simulink model "SlideMode_Control"  (R2021b)
settings: Solver=ode1  StartTime=0.0  StopTime=220  FixedStep=0.01  RelTol=1e-3
values from neighbouring files (symbols this model uses):
  AirDensity_kgpm3 = 1.225    [vehicle_controller.mat]
  BatteryCapacity_Wh = 83    [vehicle_controller.mat]
  BatteryInitialEnergy = 58.1    [vehicle_controller.mat]
  BatteryMaxVoltage_V = 96    [vehicle_controller.mat]
  BatteryVoltageCoefficient_x = [0 0.1 0.2 0.3 0.4 0.5 0.6 0.7 0.8 0.9 1]    [vehicle_controller.mat]
  BatteryVoltageCoefficient_y = [0.833333333333 0.85 0.866666666667 0.883333333333 0.9 0.916666666667 0.933333333333 0.95 0.966666666667 0.983333333333 1]    [vehicle_controller.mat]
  BodyInitialSpeed_mps = 0    [vehicle_controller.mat]
  BodyMass_kg = 900    [vehicle_controller.mat]
  CombustionEngineMaxTorque_Nm = 100    [vehicle_controller.mat]
  DragArea_m2 = 4.5    [vehicle_controller.mat]
  DragCoeficient_1 = 0.4    [vehicle_controller.mat]
  FrictionCoefficient_Nsprad = 0.01    [vehicle_controller.mat]
  GearboxRatio_0_1 = 3    [vehicle_controller.mat]
  Ke = 0.1178    [vehicle_controller.mat]
  Kt = 0.668    [vehicle_controller.mat]
  L = looptransfer.Lo    [H_infinity_control_design.m]    (also in LoopShaping.m = G*K; Vehicle_Car_Controller.m = P * C)
  R = 0.141176    [vehicle_controller.mat]
  WheelDiameter_m = 0.5    [vehicle_controller.mat]
libraries: simulink x11, simulink_extras x1, cstblocks x1
settings Model: Creator=beni  LastModifiedBy=beni
settings SolverCC: ZeroCrossAlgorithm=Adaptive
settings DataIOCC: ReturnWorkspaceOutputs=off
settings DebuggingCC: IgnoredZcDiagnostic=none

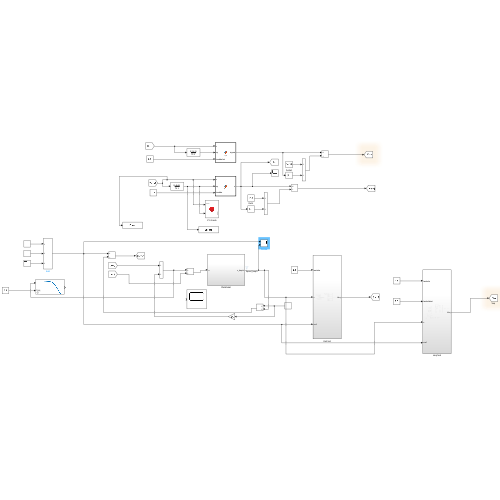
[thumbnail: Simulink's stored preview of the top-level diagram]
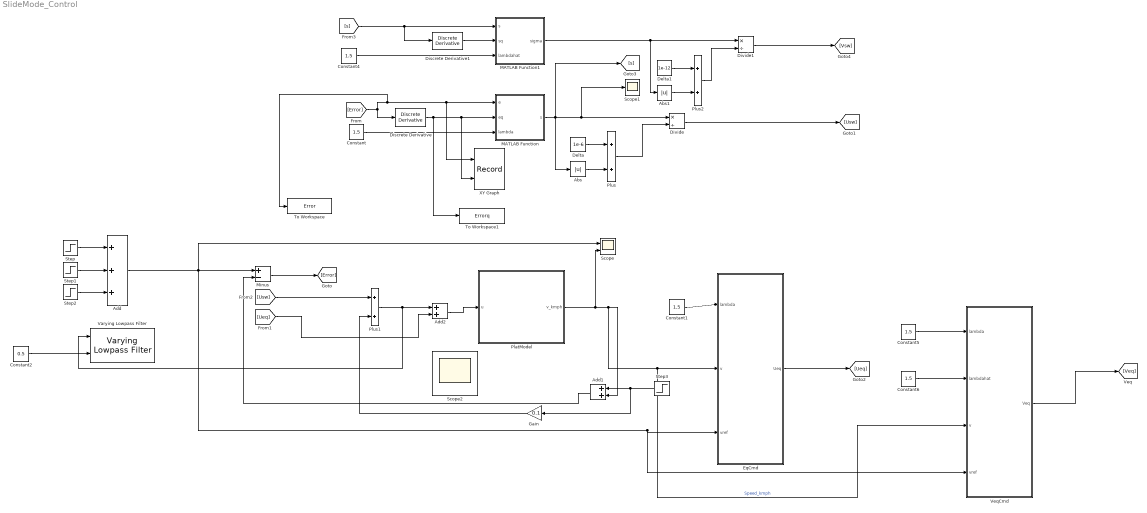
== system SlideMode_Control ==
  Abs : Abs
  Abs1 : Abs
  Add : Sum  Inputs=+++
  Add1 : Sum
  Add2 : Sum
  Constant{,1,4..6} (5 alike) : Constant  Value=1.5
  Constant2 : Constant  Value=0.5
  Delta : Constant  Value=1e-6
  Delta1 : Constant  Value=1e-12
  Discrete Derivative : simulink/Discrete/Discrete Derivative  gainval=1.0  ICPrevScaledInput=0.0  OutMin=[]  OutMax=[]  OutDataType=fixdt(1, 16)  OutScaling=2^-10  DoSatur=off
  Discrete Derivative1 : simulink/Discrete/Discrete Derivative  gainval=1.0  ICPrevScaledInput=0.0  OutMin=[]  OutMax=[]  OutDataType=fixdt(1, 16)  OutScaling=2^-10  DoSatur=off
  Divide : Product  Inputs=*/
  Divide1 : Product  Inputs=*/
  EqCmd : Subsystem
  Gain : Gain  Gain=0.1
  MATLAB Function : MATLAB Function  TreatAsAtomicUnit=on
  MATLAB Function1 : MATLAB Function  TreatAsAtomicUnit=on
  Minus : Sum  Inputs=+-
  PlatModel : Subsystem
  Plus : Sum
  Plus1 : Sum
  Plus2 : Sum
  Scope : Scope  NumInputPorts=2
  Scope1 : Scope
  Scope2 : Scope
  Step : Step  After=63  SampleTime=0
  Step1 : Step  Time=100  After=75  SampleTime=0
  Step2 : Step  Time=150  After=-20  SampleTime=0
  Step3 : Step  Time=40  After=5  SampleTime=0
  To Workspace : ToWorkspace  VariableName=Error  SampleTime=-1
  To Workspace1 : ToWorkspace  VariableName=Errorq  SampleTime=-1
  Varying Lowpass Filter : cstblocks/Linear Parameter Varying/Varying Lowpass Filter  N=1
  VeqCmd : Subsystem
  XY Graph : Record  FileSettingsInternal="{\"entries\":[{\"content\":{\"excelSettings\":{\"content\":{},\"type\":\"Streamout.ExcelSettings\"}},\"type\":\"Streamout.FileSettingStorage\",\"uuid\":\"e4c54855-29c5-47fe-8363-1f54683a9ba0\"}],\"packageUris\":[\"http://schema.mathworks.com/mf0/streamout_blocks/R2020a\"],\"version\":\"1.0\"}"  Layout=[1 1]  SignalsInternal="{\"entries\":[{\"content\":{\"signals\":[{\"content\":{\"blockPath\":[\"SlideMode_Control/XY Graph\"],\"channel\":[],\"dimensions\":[1],\"domain\":\"SlideMode_Control/XY Graph\",\"lineColor\":\"#a2142f\",\"plots\":[],\"port\":1,\"sid\":[\"\"],\"signalID\":7298,\"signalName\":\"From\"},\"type\":\"RecordBlkView.Signal\",\"uuid\":\"8499915c-e861-4faa-950b-0bc3fc22a372\"},{\"content\":{\"blockPath\":[\"SlideMode_Control/XY Graph\"],\"channel\":[],\"dimensions\":[1],\"domain\":\"SlideMode_Control/XY Graph\",\"lineColor\":\"#139fff\",\"plots\":[1],\"port\":2,\"sid\":[\"\"],\"signalID\":7302,\"signalName\":\"Discrete Derivative\"},\"type\":\"RecordBlkView.Signal\",\"uuid\":\"a22b5c38-c1a7-44f1-81eb-330b2b590f18\"}]},\"type\":\"RecordBlkView.InputSignals\",\"uuid\":\"09383715-5c63-4da3-889c-474507ecce84\"}],\"packageUris\":[\"http://schema.mathworks.com/mf0/streamout_blocks/R2020a\"],\"version\":\"1.0\"}"  VisualizationBindings="{\"xyplotplugin\":{\"info\":[{\"series\":[{\"bindingParametersList\":[{\"parameter\":\"Y-Axis\",\"signalID\":7302,\"signalName\":\"Discrete Derivative\"}],\"seriesID\":63923}],\"subplotID\":1}]}}"  CompatibilityTag=XY
  wires:
  PlatModel/1(v_kmph) -> Scope/2, Add1/2, VeqCmd/3(v), EqCmd/2(v)  "Speed_kmph"
  Minus/1 -> [Error]
  [Error] -> Discrete Derivative/1, To Workspace/1, XY Graph/1, MATLAB Function/1(e)
  Discrete Derivative/1 -> To Workspace1/1, XY Graph/2, MATLAB Function/2(eq)
  Constant/1 -> MATLAB Function/3(lambda)
  Abs/1 -> Plus/2
  MATLAB Function/1(s) -> [s], Scope1/1, Divide/1, Abs/1
  Delta/1 -> Plus/1
  Plus/1 -> Divide/2
  Constant1/1 -> EqCmd/1(lambda)
  EqCmd/1(Ueq) -> [Ueq]
  [Usw] -> Plus1/1
  Divide/1 -> [Usw]
  Constant2/1 -> Varying Lowpass Filter/2
  VeqCmd/1(Veq) -> [Veq]
  Discrete Derivative1/1 -> MATLAB Function1/2(sq)
  [s] -> Discrete Derivative1/1, MATLAB Function1/1(s)
  Constant4/1 -> MATLAB Function1/3(lambdahat)
  Delta1/1 -> Plus2/1
  Plus2/1 -> Divide1/2
  MATLAB Function1/1(sigma) -> Abs1/1, Divide1/1
  Divide1/1 -> [Vsw]
  Abs1/1 -> Plus2/2
  Constant5/1 -> VeqCmd/1(lambda)
  Constant6/1 -> VeqCmd/2(lambdahat)
  Plus1/1 -> Add2/1, Varying Lowpass Filter/1
  Add/1 -> Scope/1, VeqCmd/4(vref), EqCmd/3(vref), Minus/1
  Add1/1 -> Minus/2
  Step/1 -> Add/1
  Step1/1 -> Add/2
  Step2/1 -> Add/3
  Step3/1 -> Gain/1, Add1/1
  Add2/1 -> PlatModel/1(u)
  Gain/1 -> Plus1/2
  [Ueq] -> Add2/2

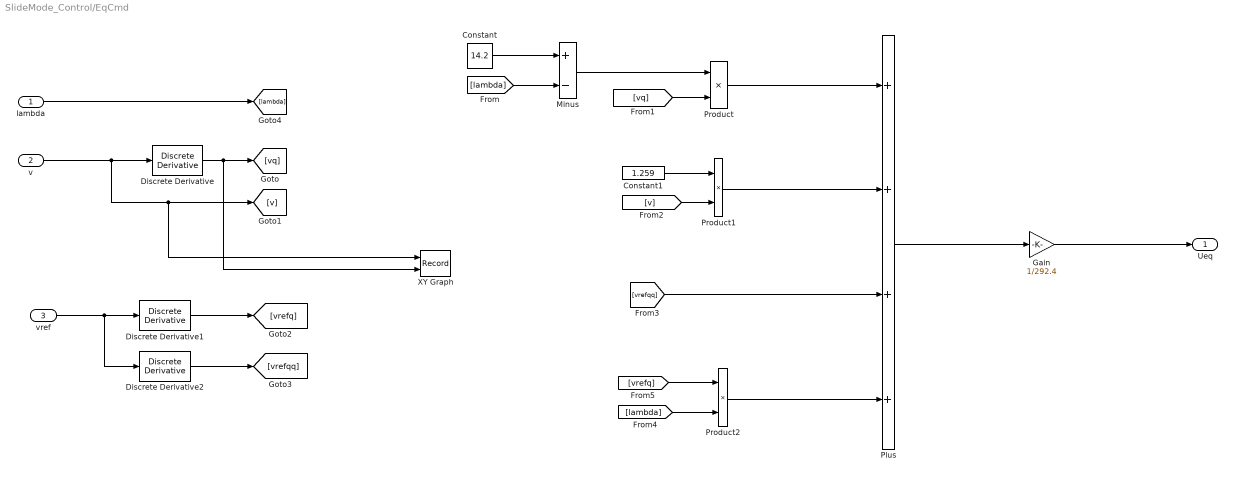
== system SlideMode_Control/EqCmd ==
  lambda : Inport
  v : Inport  Port=2
  vref : Inport  Port=3
  Constant : Constant  Value=14.2
  Constant1 : Constant  Value=1.259
  Discrete Derivative : simulink/Discrete/Discrete Derivative  gainval=1.0  ICPrevScaledInput=0.0  OutMin=[]  OutMax=[]  OutDataType=fixdt(1, 16)  OutScaling=2^-10  DoSatur=off
  Discrete Derivative1 : simulink/Discrete/Discrete Derivative  gainval=1.0  ICPrevScaledInput=0.0  OutMin=[]  OutMax=[]  OutDataType=fixdt(1, 16)  OutScaling=2^-10  DoSatur=off
  Discrete Derivative2 : simulink/Discrete/Discrete Derivative  gainval=1.0  ICPrevScaledInput=0.0  OutMin=[]  OutMax=[]  OutDataType=fixdt(1, 16)  OutScaling=2^-10  DoSatur=off
  Gain : Gain  Gain=1/292.4
  Minus : Sum  Inputs=+-
  Plus : Sum  Inputs=++++
  Product : Product
  Product1 : Product
  Product2 : Product
  XY Graph : Record  FileSettingsInternal="{\"entries\":[{\"content\":{\"excelSettings\":{\"content\":{},\"type\":\"Streamout.ExcelSettings\"}},\"type\":\"Streamout.FileSettingStorage\",\"uuid\":\"b16a5f91-d4a1-49a2-a27a-15ddc10f0a7e\"}],\"packageUris\":[\"http://schema.mathworks.com/mf0/streamout_blocks/R2020a\"],\"version\":\"1.0\"}"  Layout=[1 1]  SignalsInternal="{\"entries\":[{\"content\":{\"signals\":[{\"content\":{\"blockPath\":[\"SlideMode_Control/EqCmd/XY Graph\"],\"channel\":[],\"dimensions\":[1],\"domain\":\"SlideMode_Control/EqCmd/XY Graph\",\"lineColor\":\"#a2142f\",\"plots\":[1],\"port\":1,\"sid\":[\"\"],\"signalID\":7314,\"signalName\":\"v\"},\"type\":\"RecordBlkView.Signal\",\"uuid\":\"f1ec4534-eb6a-4768-bd96-3897fc4c94d6\"},{\"content\":{\"blockPath\":[\"SlideMode_Control/EqCmd/XY Graph\"],\"channel\":[],\"dimensions\":[1],\"domain\":\"SlideMode_Control/EqCmd/XY Graph\",\"lineColor\":\"#139fff\",\"plots\":[1],\"port\":2,\"sid\":[\"\"],\"signalID\":7318,\"signalName\":\"Discrete Derivative\"},\"type\":\"RecordBlkView.Signal\",\"uuid\":\"f4cb1554-1745-48c5-b1b8-53c7b26e64ab\"}]},\"type\":\"RecordBlkView.InputSignals\",\"uuid\":\"a4abee9c-6360-49de-9ab9-487291d355fa\"}],\"packageUris\":[\"http://schema.mathworks.com/mf0/streamout_blocks/R2020a\"],\"version\":\"1.0\"}"  VisualizationBindings="{\"xyplotplugin\":{\"info\":[{\"series\":[{\"bindingParametersList\":[{\"parameter\":\"X-Axis\",\"signalID\":7314,\"signalName\":\"v\"},{\"parameter\":\"Y-Axis\",\"signalID\":7318,\"signalName\":\"Discrete Derivative\"}],\"seriesID\":11742}],\"subplotID\":1}]}}"  CompatibilityTag=XY
  Ueq : Outport
  wires:
  v/1 -> Discrete Derivative/1, XY Graph/1, [v]
  Discrete Derivative/1 -> XY Graph/2, [vq]
  vref/1 -> Discrete Derivative2/1, Discrete Derivative1/1
  Discrete Derivative1/1 -> [vrefq]
  Discrete Derivative2/1 -> [vrefqq]
  lambda/1 -> [lambda]
  Constant/1 -> Minus/1
  [lambda] -> Minus/2
  Minus/1 -> Product/1
  [vq] -> Product/2
  Product/1 -> Plus/1
  Constant1/1 -> Product1/1
  [v] -> Product1/2
  Product1/1 -> Plus/2
  [vrefqq] -> Plus/3
  Product2/1 -> Plus/4
  [lambda] -> Product2/2
  [vrefq] -> Product2/1
  Plus/1 -> Gain/1
  Gain/1 -> Ueq/1

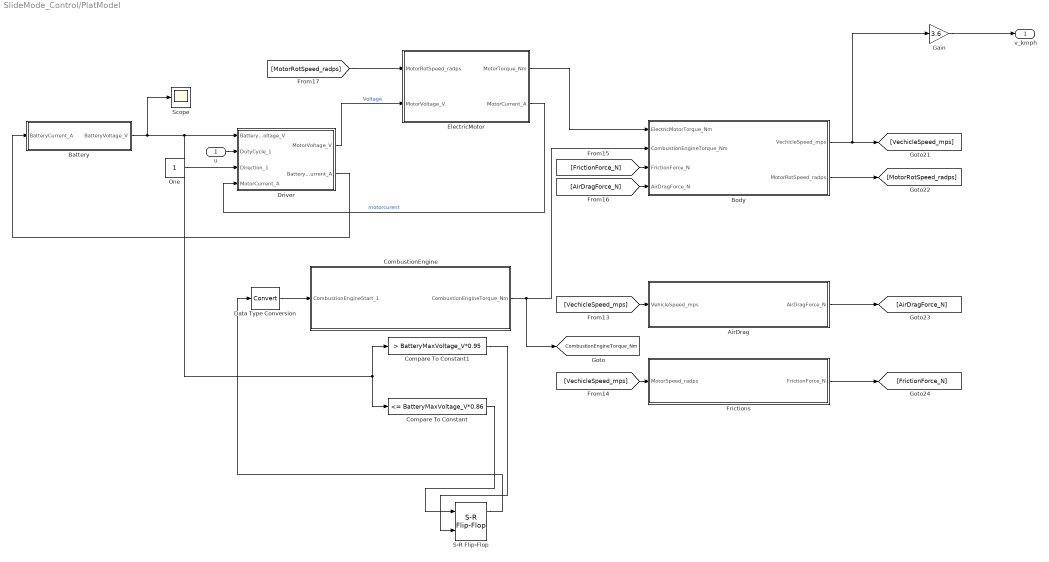
== system SlideMode_Control/PlatModel ==
  u : Inport
  AirDrag : Subsystem
  Battery : Subsystem
  Body : Subsystem
  CombustionEngine : Subsystem
  Compare To Constant : simulink/Logic and Bit Operations/Compare To Constant  relop=<=  const=BatteryMaxVoltage_V*0.86  OutDataTypeStr=boolean
  Compare To Constant1 : simulink/Logic and Bit Operations/Compare To Constant  relop=>  const=BatteryMaxVoltage_V*0.95  OutDataTypeStr=boolean
  Data Type Conversion : DataTypeConversion
  Driver : Subsystem
  ElectricMotor : Subsystem
  Frictions : Subsystem
  Gain : Gain  Gain=3.6
  One : Constant  OutDataTypeStr=Inherit: Inherit via back propagation
  S-R Flip-Flop : simulink_extras/Flip Flops/S-R Flip-Flop  initial_condition=0
  Scope : Scope
  v_kmph : Outport
  tag scope: CombustionEngineTorque_Nm=global
  wires:
  One/1 -> Driver/3(Direction_1)
  ElectricMotor/1(MotorTorque_Nm) -> Body/1(ElectricMotorTorque_Nm)
  [FrictionForce_N] -> Body/3(FrictionForce_N)
  Body/1(VechicleSpeed_mps) -> [VechicleSpeed_mps], Gain/1
  Body/2(MotorRotSpeed_radps) -> [MotorRotSpeed_radps]
  AirDrag/1(AirDragForce_N) -> [AirDragForce_N]
  Frictions/1(FrictionForce_N) -> [FrictionForce_N]
  [VechicleSpeed_mps] -> AirDrag/1(VehicleSpeed_mps)
  [AirDragForce_N] -> Body/4(AirDragForce_N)
  [MotorRotSpeed_radps] -> ElectricMotor/1(MotorRotSpeed_radps)
  [VechicleSpeed_mps] -> Frictions/1(MotorSpeed_radps)
  ElectricMotor/2(MotorCurrent_A) -> Driver/4(MotorCurrent_A)  "motorcurent"
  u/1 -> Driver/2(DutyCycle_1)
  Gain/1 -> v_kmph/1
  Data Type Conversion/1 -> CombustionEngine/1(CombustionEngineStart_1)
  CombustionEngine/1(CombustionEngineTorque_Nm) -> Body/2(CombustionEngineTorque_Nm), [CombustionEngineTorque_Nm]
  Driver/2(BatteryCurrent_A) -> Battery/1(BatteryCurrent_A)
  Driver/1(MotorVoltage_V) -> ElectricMotor/2(MotorVoltage_V)  "Voltage"
  Compare To Constant1/1 -> S-R Flip-Flop/2
  Compare To Constant/1 -> S-R Flip-Flop/1
  S-R Flip-Flop/1 -> Data Type Conversion/1
  Battery/1(BatteryVoltage_V) -> Scope/1, Driver/1(BatteryVoltage_V), Compare To Constant1/1, Compare To Constant/1

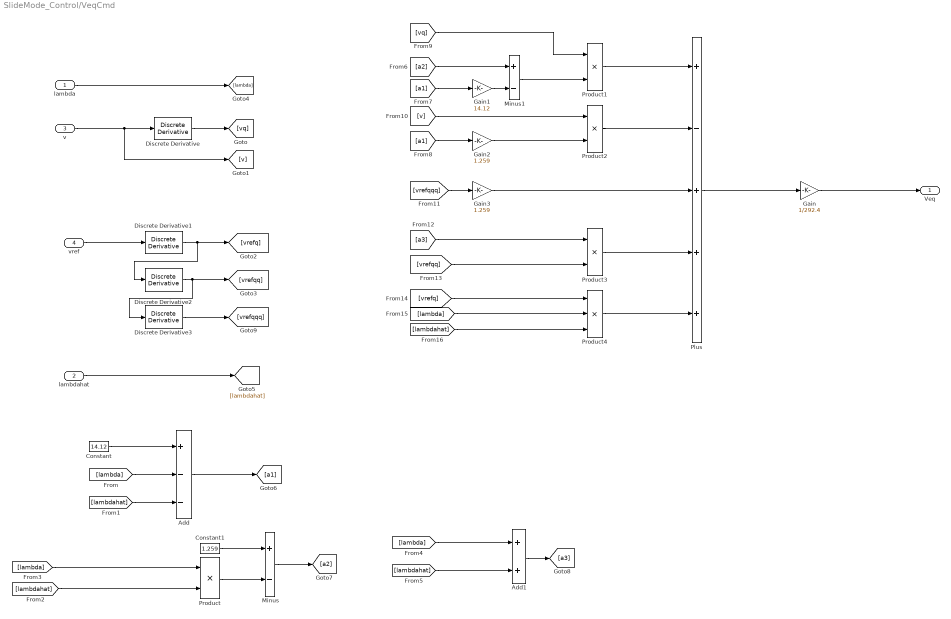
== system SlideMode_Control/VeqCmd ==
  lambda : Inport
  lambdahat : Inport  Port=2
  v : Inport  Port=3
  vref : Inport  Port=4
  Add : Sum  Inputs=+--
  Add1 : Sum
  Constant : Constant  Value=14.12
  Constant1 : Constant  Value=1.259
  Discrete Derivative{,1..3} (4 alike) : simulink/Discrete/Discrete Derivative  gainval=1.0  ICPrevScaledInput=0.0  OutMin=[]  OutMax=[]  OutDataType=fixdt(1, 16)  OutScaling=2^-10  DoSatur=off
  Gain : Gain  Gain=1/292.4
  Gain1 : Gain  Gain=14.12
  Gain2 : Gain  Gain=1.259
  Gain3 : Gain  Gain=1.259
  Minus : Sum  Inputs=+-
  Minus1 : Sum  Inputs=+-
  Plus : Sum  Inputs=+-+++
  Product{,1..3} (4 alike) : Product
  Product4 : Product  Inputs=3
  Veq : Outport
  wires:
  Gain/1 -> Veq/1
  Plus/1 -> Gain/1
  lambda/1 -> [lambda]
  Discrete Derivative2/1 -> Discrete Derivative3/1, [vrefqq]
  Discrete Derivative1/1 -> Discrete Derivative2/1, [vrefq]
  vref/1 -> Discrete Derivative1/1
  Discrete Derivative/1 -> [vq]
  v/1 -> [v], Discrete Derivative/1
  lambdahat/1 -> [lambdahat]
  Constant/1 -> Add/1
  [lambda] -> Add/2
  [lambdahat] -> Add/3
  Add/1 -> [a1]
  [lambdahat] -> Product/2
  [lambda] -> Product/1
  Product/1 -> Minus/2
  Constant1/1 -> Minus/1
  Minus/1 -> [a2]
  [lambda] -> Add1/1
  Add1/1 -> [a3]
  [lambdahat] -> Add1/2
  [a2] -> Minus1/1
  [a1] -> Gain1/1
  Gain1/1 -> Minus1/2
  [a1] -> Gain2/1
  Minus1/1 -> Product1/2
  Product1/1 -> Plus/1
  [vq] -> Product1/1
  Gain2/1 -> Product2/2
  Product2/1 -> Plus/2
  [v] -> Product2/1
  Discrete Derivative3/1 -> [vrefqqq]
  [vrefqqq] -> Gain3/1
  Gain3/1 -> Plus/3
  Product3/1 -> Plus/4
  [a3] -> Product3/1
  [vrefqq] -> Product3/2
  Product4/1 -> Plus/5
  [vrefq] -> Product4/1
  [lambda] -> Product4/2
  [lambdahat] -> Product4/3

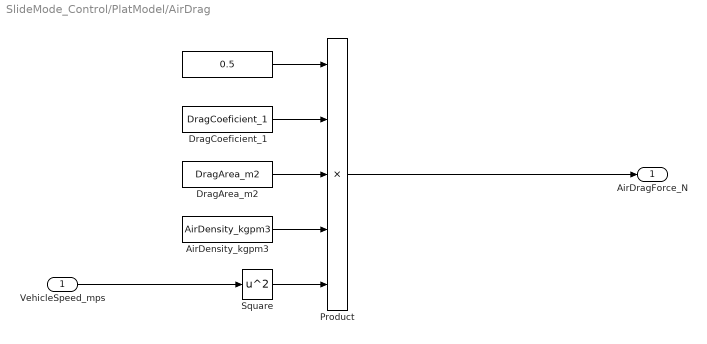
== system SlideMode_Control/PlatModel/AirDrag ==
  VehicleSpeed_mps : Inport
  " " : Constant  Value=0.5
  AirDensity_kgpm3 : Constant  Value=AirDensity_kgpm3
  DragArea_m2 : Constant  Value=DragArea_m2
  DragCoeficient_1 : Constant  Value=DragCoeficient_1
  Product : Product  Inputs=5
  Square : Math  Operator=square  SaturateOnIntegerOverflow=on
  AirDragForce_N : Outport
  wires:
  VehicleSpeed_mps/1 -> Square/1
  Square/1 -> Product/5
  DragArea_m2/1 -> Product/3
  AirDensity_kgpm3/1 -> Product/4
  DragCoeficient_1/1 -> Product/2
  " "/1 -> Product/1
  Product/1 -> AirDragForce_N/1

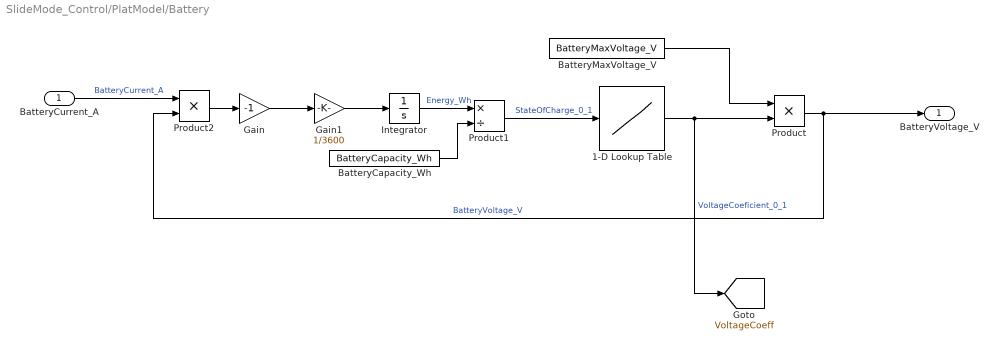
== system SlideMode_Control/PlatModel/Battery ==
  BatteryCurrent_A : Inport
  1-D Lookup Table : Lookup_n-D  NumberOfTableDimensions=1  BreakpointsForDimension1=BatteryVoltageCoefficient_x  Table=BatteryVoltageCoefficient_y  InternalRulePriority=Speed  RndMeth=Simplest  InputSameDT=on
  BatteryCapacity_Wh : Constant  Value=BatteryCapacity_Wh
  BatteryMaxVoltage_V : Constant  Value=BatteryMaxVoltage_V
  Gain : Gain  Gain=-1
  Gain1 : Gain  Gain=1/3600
  Integrator : Integrator  InitialCondition=BatteryInitialEnergy
  Product : Product
  Product1 : Product  Inputs=*/
  Product2 : Product
  BatteryVoltage_V : Outport
  tag scope: VoltageCoeff=global
  wires:
  BatteryCurrent_A/1 -> Product2/1  "BatteryCurrent_A"
  Product/1 -> Product2/2, BatteryVoltage_V/1  "BatteryVoltage_V"
  Integrator/1 -> Product1/1  "Energy_Wh"
  1-D Lookup Table/1 -> [VoltageCoeff], Product/2  "VoltageCoeficient_0_1"
  BatteryMaxVoltage_V/1 -> Product/1
  BatteryCapacity_Wh/1 -> Product1/2
  Product1/1 -> 1-D Lookup Table/1  "StateOfCharge_0_1"
  Product2/1 -> Gain/1
  Gain/1 -> Gain1/1
  Gain1/1 -> Integrator/1

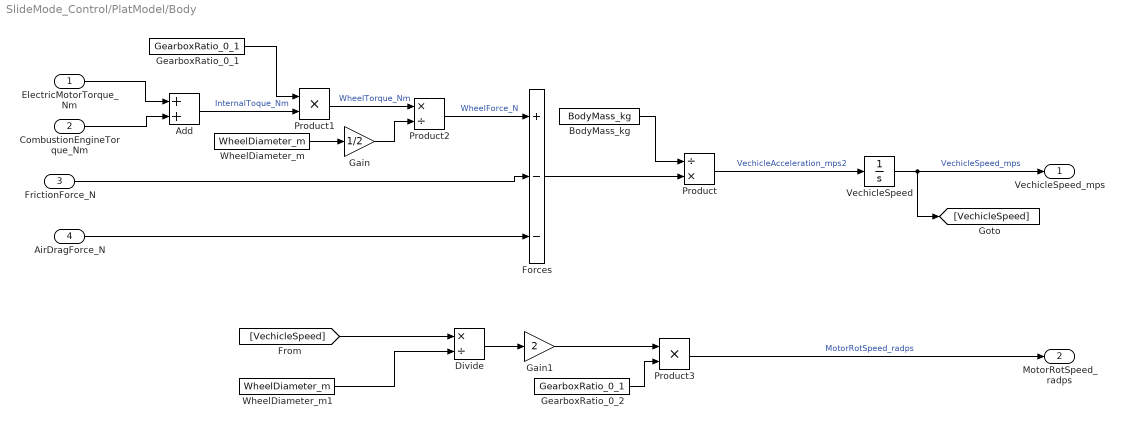
== system SlideMode_Control/PlatModel/Body ==
  ElectricMotorTorque_Nm : Inport
  CombustionEngineTorque_Nm : Inport  Port=2
  FrictionForce_N : Inport  Port=3
  AirDragForce_N : Inport  Port=4
  Add : Sum
  BodyMass_kg : Constant  Value=BodyMass_kg
  Divide : Product  Inputs=*/
  Forces : Sum  Inputs=+--
  Gain : Gain  Gain=1/2
  Gain1 : Gain  Gain=2
  GearboxRatio_0_1 : Constant  Value=GearboxRatio_0_1
  GearboxRatio_0_2 : Constant  Value=GearboxRatio_0_1
  Product : Product  Inputs=/*
  Product1 : Product
  Product2 : Product  Inputs=*/
  Product3 : Product  Inputs=**
  VechicleSpeed : Integrator  InitialCondition=BodyInitialSpeed_mps
  WheelDiameter_m : Constant  Value=WheelDiameter_m
  WheelDiameter_m1 : Constant  Value=WheelDiameter_m
  VechicleSpeed_mps : Outport
  MotorRotSpeed_radps : Outport  Port=2
  wires:
  VechicleSpeed/1 -> [VechicleSpeed], VechicleSpeed_mps/1  "VechicleSpeed_mps"
  Product/1 -> VechicleSpeed/1  "VechicleAcceleration_mps2"
  BodyMass_kg/1 -> Product/1
  Forces/1 -> Product/2
  AirDragForce_N/1 -> Forces/3
  FrictionForce_N/1 -> Forces/2
  ElectricMotorTorque_Nm/1 -> Add/1
  CombustionEngineTorque_Nm/1 -> Add/2
  Add/1 -> Product1/2  "InternalToque_Nm"
  GearboxRatio_0_1/1 -> Product1/1
  Product1/1 -> Product2/1  "WheelTorque_Nm"
  WheelDiameter_m/1 -> Gain/1
  Product2/1 -> Forces/1  "WheelForce_N"
  Gain/1 -> Product2/2
  [VechicleSpeed] -> Divide/1
  WheelDiameter_m1/1 -> Divide/2
  Divide/1 -> Gain1/1
  Gain1/1 -> Product3/1
  GearboxRatio_0_2/1 -> Product3/2
  Product3/1 -> MotorRotSpeed_radps/1  "MotorRotSpeed_radps"

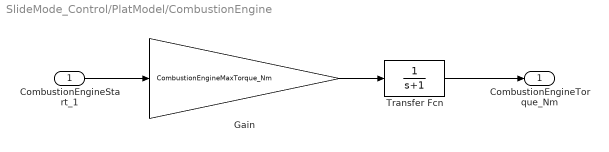
== system SlideMode_Control/PlatModel/CombustionEngine ==
  CombustionEngineStart_1 : Inport
  Gain : Gain  Gain=CombustionEngineMaxTorque_Nm
  Transfer Fcn : TransferFcn  Denominator=[1 1]
  CombustionEngineTorque_Nm : Outport
  wires:
  Transfer Fcn/1 -> CombustionEngineTorque_Nm/1
  CombustionEngineStart_1/1 -> Gain/1
  Gain/1 -> Transfer Fcn/1

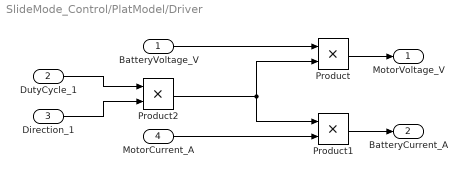
== system SlideMode_Control/PlatModel/Driver ==
  BatteryVoltage_V : Inport
  DutyCycle_1 : Inport  Port=2
  Direction_1 : Inport  Port=3
  MotorCurrent_A : Inport  Port=4
  Product : Product
  Product1 : Product
  Product2 : Product
  MotorVoltage_V : Outport
  BatteryCurrent_A : Outport  Port=2
  wires:
  BatteryVoltage_V/1 -> Product/1
  Product/1 -> MotorVoltage_V/1
  Product2/1 -> Product1/1, Product/2
  MotorCurrent_A/1 -> Product1/2
  Product1/1 -> BatteryCurrent_A/1
  DutyCycle_1/1 -> Product2/1
  Direction_1/1 -> Product2/2

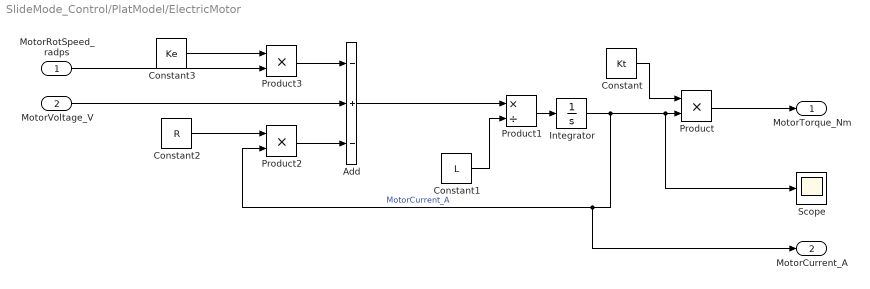
== system SlideMode_Control/PlatModel/ElectricMotor ==
  MotorRotSpeed_radps : Inport
  MotorVoltage_V : Inport  Port=2
  Add : Sum  Inputs=-+-
  Constant : Constant  Value=Kt
  Constant1 : Constant  Value=L
  Constant2 : Constant  Value=R
  Constant3 : Constant  Value=Ke
  Integrator : Integrator
  Product : Product
  Product1 : Product  Inputs=*/
  Product2 : Product
  Product3 : Product
  Scope : Scope
  MotorTorque_Nm : Outport
  MotorCurrent_A : Outport  Port=2
  wires:
  Product/1 -> MotorTorque_Nm/1
  Integrator/1 -> MotorCurrent_A/1, Product2/2, Scope/1, Product/2  "MotorCurrent_A"
  Constant/1 -> Product/1
  Product1/1 -> Integrator/1
  Constant1/1 -> Product1/2
  Add/1 -> Product1/1
  Product2/1 -> Add/3
  Constant2/1 -> Product2/1
  MotorVoltage_V/1 -> Add/2
  Constant3/1 -> Product3/1
  Product3/1 -> Add/1
  MotorRotSpeed_radps/1 -> Product3/2

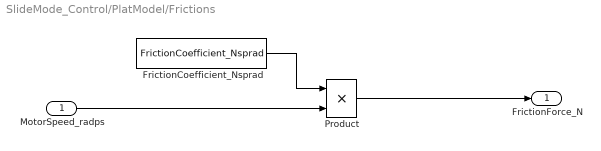
== system SlideMode_Control/PlatModel/Frictions ==
  MotorSpeed_radps : Inport
  FrictionCoefficient_Nsprad : Constant  Value=FrictionCoefficient_Nsprad
  Product : Product
  FrictionForce_N : Outport
  wires:
  Product/1 -> FrictionForce_N/1
  MotorSpeed_radps/1 -> Product/2
  FrictionCoefficient_Nsprad/1 -> Product/1

== matlab function SlideMode_Control/MATLAB Function ==
  data: e input; s output; eq input; lambda input
function s = fcn(e,eq,lambda)

s = lambda*e + eq;

end

== matlab function SlideMode_Control/MATLAB Function1 ==
  data: s input; sigma output; sq input; lambdahat input
function sigma = fcn(s,sq,lambdahat)

sigma = lambdahat*s + sq;

end
